simulink library "avlAerodynamics"  (R2018b)
settings: Solver=VariableStepAuto  StartTime=0.0  StopTime=10.0  RelTol=1e-3
values from neighbouring files (symbols this model uses):
  refArea = 1    [avlAerodynamics_ts.m]
undefined symbols (not defined in the file or in its folder): CLtotTbl
libraries: alphaBeta_ul x1
settings Model: Creator=mcobb  LastModifiedBy=mcobb

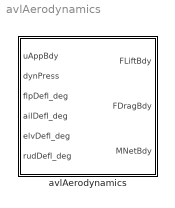
== system avlAerodynamics ==
  avlAerodynamics : Subsystem  mask{CLTable=CLtotTbl, CDTable=CLtotTbl, CMxTable=CLtotTbl, CMyTable=CLtotTbl, CMzTable=CLtotTbl, SRef=0, BRef=0, CRef=0}
      mask prompts: CLTable "CL lookup table object"; CDTable "CD lookup table object"; CMxTable "CMx lookup table object"; CMyTable "CMy lookup table object"; CMzTable "CMz lookup table object"; SRef "Ref area (AVL Sref)"; BRef "Roll & Yaw Moment Reference Length (AVL Bref)"; CRef "Pitch Moment Reference Length (AVL Cref)"
      mask DialogControl Container4 Prompt: Reference Areas

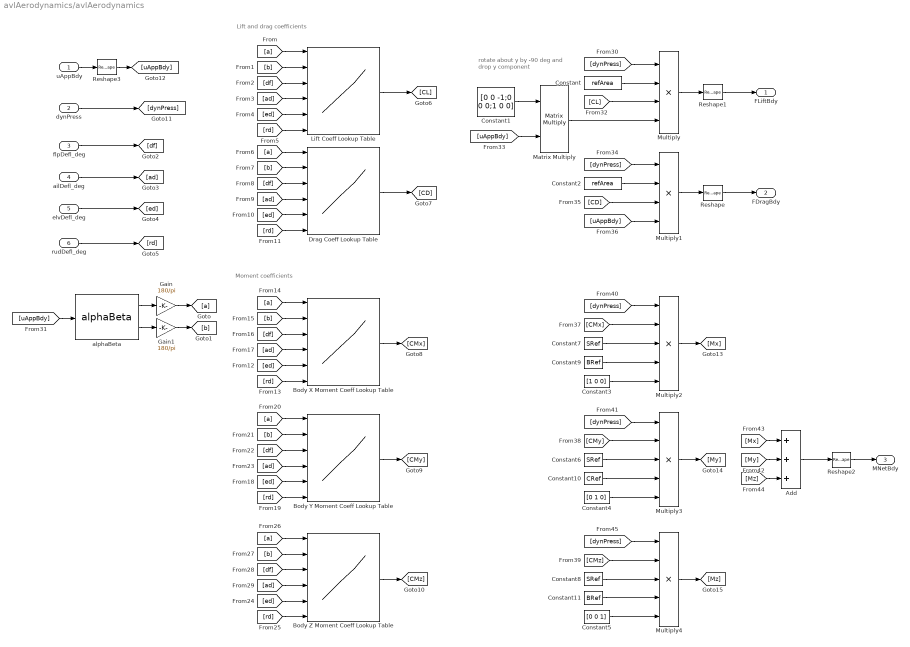
== system avlAerodynamics/avlAerodynamics ==
  note: rotate about y by -90 deg
      | and drop y component
  note: Moment coefficients
  note: Lift and drag coefficients
  uAppBdy : Inport
  dynPress : Inport  Port=2
  flpDefl_deg : Inport  Port=3
  ailDefl_deg : Inport  Port=4
  elvDefl_deg : Inport  Port=5
  rudDefl_deg : Inport  Port=6
  Add : Sum  Inputs=+++
  Body X Moment Coeff Lookup Table : Lookup_n-D  NumberOfTableDimensions=6  DataSpecification=Lookup table object  LookupTableObject=CMxTable  BreakpointsForDimension3=[5, 7]  Table=reshape(repmat([4 5 6;16 19 20;10 18 23],1,2),[3,3,2])  InternalRulePriority=Speed  RndMeth=Simplest  InputSameDT=on
  Body Y Moment Coeff Lookup Table : Lookup_n-D  NumberOfTableDimensions=6  DataSpecification=Lookup table object  LookupTableObject=CMyTable  BreakpointsForDimension3=[5, 7]  Table=reshape(repmat([4 5 6;16 19 20;10 18 23],1,2),[3,3,2])  InternalRulePriority=Speed  RndMeth=Simplest  InputSameDT=on
  Body Z Moment Coeff Lookup Table : Lookup_n-D  NumberOfTableDimensions=6  DataSpecification=Lookup table object  LookupTableObject=CMzTable  BreakpointsForDimension3=[5, 7]  Table=reshape(repmat([4 5 6;16 19 20;10 18 23],1,2),[3,3,2])  InternalRulePriority=Speed  RndMeth=Simplest  InputSameDT=on
  Constant : Constant  Value=refArea
  Constant1 : Constant  Value=[0 0 -1;0 0 0;1 0 0]
  Constant10 : Constant  Value=CRef
  Constant11 : Constant  Value=BRef
  Constant2 : Constant  Value=refArea
  Constant3 : Constant  Value=[1 0 0]
  Constant4 : Constant  Value=[0 1 0]
  Constant5 : Constant  Value=[0 0 1]
  Constant6 : Constant  Value=SRef
  Constant7 : Constant  Value=SRef
  Constant8 : Constant  Value=SRef
  Constant9 : Constant  Value=BRef
  Drag Coeff Lookup Table : Lookup_n-D  NumberOfTableDimensions=6  DataSpecification=Lookup table object  LookupTableObject=CDTable  BreakpointsForDimension3=[5, 7]  Table=reshape(repmat([4 5 6;16 19 20;10 18 23],1,2),[3,3,2])  InternalRulePriority=Speed  RndMeth=Simplest  InputSameDT=on
  Gain : Gain  Gain=180/pi
  Gain1 : Gain  Gain=180/pi
  Lift Coeff Lookup Table : Lookup_n-D  NumberOfTableDimensions=6  DataSpecification=Lookup table object  LookupTableObject=CLTable  BreakpointsForDimension3=[5, 7]  Table=reshape(repmat([4 5 6;16 19 20;10 18 23],1,2),[3,3,2])  InternalRulePriority=Speed  RndMeth=Simplest  InputSameDT=on
  Matrix Multiply : Product  Multiplication=Matrix(*)
  Multiply : Product  Inputs=4
  Multiply1 : Product  Inputs=4
  Multiply2 : Product  Inputs=5
  Multiply3 : Product  Inputs=5
  Multiply4 : Product  Inputs=5
  Reshape{,1..3} (4 alike) : Reshape  OutputDimensionality=Column vector (2-D)
  alphaBeta : alphaBeta_ul/alphaBeta  SystemSampleTime=-1
  FLiftBdy : Outport
  FDragBdy : Outport  Port=2
  MNetBdy : Outport  Port=3
  wires:
  uAppBdy/1 -> Reshape3/1
  flpDefl_deg/1 -> [df]
  ailDefl_deg/1 -> [ad]
  elvDefl_deg/1 -> [ed]
  rudDefl_deg/1 -> [rd]
  [b] -> Lift Coeff Lookup Table/2
  [a] -> Lift Coeff Lookup Table/1
  [df] -> Lift Coeff Lookup Table/3
  [ad] -> Lift Coeff Lookup Table/4
  [ed] -> Lift Coeff Lookup Table/5
  [rd] -> Lift Coeff Lookup Table/6
  Lift Coeff Lookup Table/1 -> [CL]
  [rd] -> Drag Coeff Lookup Table/6
  [ed] -> Drag Coeff Lookup Table/5
  [ad] -> Drag Coeff Lookup Table/4
  [df] -> Drag Coeff Lookup Table/3
  [a] -> Drag Coeff Lookup Table/1
  [b] -> Drag Coeff Lookup Table/2
  [b] -> Body X Moment Coeff Lookup Table/2
  [a] -> Body X Moment Coeff Lookup Table/1
  [df] -> Body X Moment Coeff Lookup Table/3
  [ad] -> Body X Moment Coeff Lookup Table/4
  [ed] -> Body X Moment Coeff Lookup Table/5
  [rd] -> Body X Moment Coeff Lookup Table/6
  [rd] -> Body Y Moment Coeff Lookup Table/6
  [ed] -> Body Y Moment Coeff Lookup Table/5
  [ad] -> Body Y Moment Coeff Lookup Table/4
  [df] -> Body Y Moment Coeff Lookup Table/3
  [a] -> Body Y Moment Coeff Lookup Table/1
  [b] -> Body Y Moment Coeff Lookup Table/2
  [b] -> Body Z Moment Coeff Lookup Table/2
  [a] -> Body Z Moment Coeff Lookup Table/1
  [df] -> Body Z Moment Coeff Lookup Table/3
  [ad] -> Body Z Moment Coeff Lookup Table/4
  [ed] -> Body Z Moment Coeff Lookup Table/5
  [rd] -> Body Z Moment Coeff Lookup Table/6
  Drag Coeff Lookup Table/1 -> [CD]
  Body X Moment Coeff Lookup Table/1 -> [CMx]
  Body Y Moment Coeff Lookup Table/1 -> [CMy]
  Body Z Moment Coeff Lookup Table/1 -> [CMz]
  alphaBeta/1 -> Gain/1
  alphaBeta/2 -> Gain1/1
  Gain/1 -> [a]
  Gain1/1 -> [b]
  dynPress/1 -> [dynPress]
  [uAppBdy] -> alphaBeta/1
  [dynPress] -> Multiply/1
  Constant/1 -> Multiply/2
  [CL] -> Multiply/3
  Matrix Multiply/1 -> Multiply/4
  Constant1/1 -> Matrix Multiply/1
  [uAppBdy] -> Matrix Multiply/2
  [CD] -> Multiply1/3
  Constant2/1 -> Multiply1/2
  [dynPress] -> Multiply1/1
  [uAppBdy] -> Multiply1/4
  Multiply/1 -> Reshape1/1
  Multiply1/1 -> Reshape/1
  Reshape1/1 -> FLiftBdy/1
  Reshape/1 -> FDragBdy/1
  [CMx] -> Multiply2/2
  Multiply2/1 -> [Mx]
  Multiply3/1 -> [My]
  [CMy] -> Multiply3/2
  [CMz] -> Multiply4/2
  Multiply4/1 -> [Mz]
  [My] -> Add/2
  [Mx] -> Add/1
  [Mz] -> Add/3
  Add/1 -> Reshape2/1
  Reshape2/1 -> MNetBdy/1
  Reshape3/1 -> [uAppBdy]
  Constant7/1 -> Multiply2/3
  Constant6/1 -> Multiply3/3
  Constant8/1 -> Multiply4/3
  Constant3/1 -> Multiply2/5
  Constant4/1 -> Multiply3/5
  Constant5/1 -> Multiply4/5
  [dynPress] -> Multiply3/1
  [dynPress] -> Multiply4/1
  Constant9/1 -> Multiply2/4
  [dynPress] -> Multiply2/1
  Constant10/1 -> Multiply3/4
  Constant11/1 -> Multiply4/4
